simulink model "gm_sampleModel61442_pp_12_1_sub"  (R2023b)
settings: Solver=VariableStepAuto  StartTime=0.0  StopTime=10.0  RelTol=1e-3
libraries: simulink x37
(part 2 of 2)

== system gm_sampleModel61442_pp_12_1_sub/Subsystem/cfblk71 ==
  emi_243 : Inport  OutDataTypeStr=uint8  PortDimensions=1  SampleTime=1
  Action Port : Inport  Port=2  OutDataTypeStr=boolean  SampleTime=1
  Reshape : Reshape
  cfblk71_out1bypassMux : MultiPortSwitch  DataPortOrder=Zero-based contiguous  Inputs=2  zeroidx=on  OutDataTypeStr=uint8  SampleTime=1  SaturateOnIntegerOverflow=off  InputSameDT=off
  emi_244_bypass : UnitDelay  InitialCondition="fi(0,0,8,0,\"hex\",\"00\")"  SampleTime=1
  emi_244 : Outport  SampleTime=1  InitialOutput=0
  wires:
  Action Port/1 -> cfblk71_out1bypassMux/1
  emi_243/1 -> Reshape/1
  Reshape/1 -> cfblk71_out1bypassMux/3
  cfblk71_out1bypassMux/1 -> emi_244_bypass/1, emi_244/1
  emi_244_bypass/1 -> cfblk71_out1bypassMux/2

== system gm_sampleModel61442_pp_12_1_sub/Subsystem/cfblk72 ==
  emi_251 : Inport  OutDataTypeStr=uint8  PortDimensions=1  SampleTime=1
  Action Port : Inport  Port=2  OutDataTypeStr=boolean  SampleTime=1
  cfblk72 : MinMax
  cfblk72_out1bypassMux : MultiPortSwitch  DataPortOrder=Zero-based contiguous  Inputs=2  zeroidx=on  OutDataTypeStr=uint8  SampleTime=1  SaturateOnIntegerOverflow=off  InputSameDT=off
  emi_252_bypass : UnitDelay  InitialCondition="fi(0,0,8,0,\"hex\",\"00\")"  SampleTime=1
  emi_252 : Outport  SampleTime=1  InitialOutput=0
  wires:
  Action Port/1 -> cfblk72_out1bypassMux/1
  emi_251/1 -> cfblk72/1
  cfblk72/1 -> cfblk72_out1bypassMux/3
  cfblk72_out1bypassMux/1 -> emi_252_bypass/1, emi_252/1
  emi_252_bypass/1 -> cfblk72_out1bypassMux/2

== system gm_sampleModel61442_pp_12_1_sub/Subsystem/cfblk75_inst ==
  in1 : Inport  OutDataTypeStr=uint8  SampleTime=1
  in2 : Inport  Port=2  OutDataTypeStr=uint8  SampleTime=1
  mul_cfblk75_dotp_mulcomp : Product  Inputs=**  OutDataTypeStr=uint8  SampleTime=1
  out1 : Outport  OutDataTypeStr=uint8  SampleTime=1
  wires:
  in1/1 -> mul_cfblk75_dotp_mulcomp/1
  in2/1 -> mul_cfblk75_dotp_mulcomp/2
  mul_cfblk75_dotp_mulcomp/1 -> out1/1

== system gm_sampleModel61442_pp_12_1_sub/Subsystem/cfblk77 ==
  emi_259 : Inport  OutDataTypeStr=uint8  PortDimensions=1  SampleTime=1
  Action Port : Inport  Port=2  OutDataTypeStr=boolean  SampleTime=1
  cfblk77 : Subsystem  mask(Real World Value Increment){}
      mask help: Simulink:masks:RealWorldValueIncrement_MD
      mask Display: disp('V++')
  cfblk77_out1bypassMux : MultiPortSwitch  DataPortOrder=Zero-based contiguous  Inputs=2  zeroidx=on  OutDataTypeStr=uint8  SampleTime=1  SaturateOnIntegerOverflow=off  InputSameDT=off
  emi_260_bypass : UnitDelay  InitialCondition="fi(0,0,8,0,\"hex\",\"00\")"  SampleTime=1
  emi_260 : Outport  SampleTime=1  InitialOutput=0
  wires:
  Action Port/1 -> cfblk77_out1bypassMux/1
  emi_259/1 -> cfblk77/1(u)
  cfblk77/1(y) -> cfblk77_out1bypassMux/3
  cfblk77_out1bypassMux/1 -> emi_260_bypass/1, emi_260/1
  emi_260_bypass/1 -> cfblk77_out1bypassMux/2

== system gm_sampleModel61442_pp_12_1_sub/Subsystem/cfblk78 ==
  emi_131 : Inport  OutDataTypeStr=uint8  PortDimensions=1  SampleTime=1
  Action Port : Inport  Port=2  OutDataTypeStr=boolean  SampleTime=1
  cfblk78 : Signum  SampleTime=1
  cfblk78_out1bypassMux : MultiPortSwitch  DataPortOrder=Zero-based contiguous  Inputs=2  zeroidx=on  OutDataTypeStr=uint8  SampleTime=1  SaturateOnIntegerOverflow=off  InputSameDT=off
  emi_132_bypass : UnitDelay  InitialCondition="fi(0,0,8,0,\"hex\",\"00\")"  SampleTime=1
  emi_132 : Outport  SampleTime=1  InitialOutput=0
  wires:
  Action Port/1 -> cfblk78_out1bypassMux/1
  emi_131/1 -> cfblk78/1
  cfblk78/1 -> cfblk78_out1bypassMux/3
  cfblk78_out1bypassMux/1 -> emi_132_bypass/1, emi_132/1
  emi_132_bypass/1 -> cfblk78_out1bypassMux/2

== system gm_sampleModel61442_pp_12_1_sub/Subsystem/cfblk79 ==
  emi_267 : Inport  OutDataTypeStr=uint8  PortDimensions=1  SampleTime=1
  Action Port : Inport  Port=2  OutDataTypeStr=boolean  SampleTime=1
  cfblk79 : MinMax
  cfblk79_out1bypassMux : MultiPortSwitch  DataPortOrder=Zero-based contiguous  Inputs=2  zeroidx=on  OutDataTypeStr=uint8  SampleTime=1  SaturateOnIntegerOverflow=off  InputSameDT=off
  emi_268_bypass : UnitDelay  InitialCondition="fi(0,0,8,0,\"hex\",\"00\")"  SampleTime=1
  emi_268 : Outport  SampleTime=1  InitialOutput=0
  wires:
  Action Port/1 -> cfblk79_out1bypassMux/1
  emi_267/1 -> cfblk79/1
  cfblk79/1 -> cfblk79_out1bypassMux/3
  cfblk79_out1bypassMux/1 -> emi_268_bypass/1, emi_268/1
  emi_268_bypass/1 -> cfblk79_out1bypassMux/2

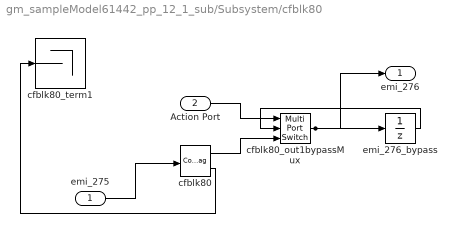
== system gm_sampleModel61442_pp_12_1_sub/Subsystem/cfblk80 ==
  emi_275 : Inport  OutDataTypeStr=uint8  PortDimensions=1  SampleTime=1
  Action Port : Inport  Port=2  OutDataTypeStr=boolean  SampleTime=1
  cfblk80 : ComplexToRealImag  SampleTime=1
  cfblk80_out1bypassMux : MultiPortSwitch  DataPortOrder=Zero-based contiguous  Inputs=2  zeroidx=on  OutDataTypeStr=uint8  SampleTime=1  SaturateOnIntegerOverflow=off  InputSameDT=off
  cfblk80_term1 : Terminator
  emi_276_bypass : UnitDelay  InitialCondition="fi(0,0,8,0,\"hex\",\"00\")"  SampleTime=1
  emi_276 : Outport  SampleTime=1  InitialOutput=0
  wires:
  Action Port/1 -> cfblk80_out1bypassMux/1
  emi_275/1 -> cfblk80/1
  cfblk80/1 -> cfblk80_out1bypassMux/3
  cfblk80/2 -> cfblk80_term1/1
  cfblk80_out1bypassMux/1 -> emi_276_bypass/1, emi_276/1
  emi_276_bypass/1 -> cfblk80_out1bypassMux/2

== system gm_sampleModel61442_pp_12_1_sub/Subsystem/cfblk81 ==
  emi_284 : Inport  OutDataTypeStr=uint8  PortDimensions=1  SampleTime=1
  Action Port : Inport  Port=2  OutDataTypeStr=boolean  SampleTime=1
  cfblk81 : MinMax
  cfblk81_out1bypassMux : MultiPortSwitch  DataPortOrder=Zero-based contiguous  Inputs=2  zeroidx=on  OutDataTypeStr=uint8  SampleTime=1  SaturateOnIntegerOverflow=off  InputSameDT=off
  emi_285_bypass : UnitDelay  InitialCondition="fi(0,0,8,0,\"hex\",\"00\")"  SampleTime=1
  emi_285 : Outport  SampleTime=1  InitialOutput=0
  wires:
  Action Port/1 -> cfblk81_out1bypassMux/1
  emi_284/1 -> cfblk81/1
  cfblk81/1 -> cfblk81_out1bypassMux/3
  cfblk81_out1bypassMux/1 -> emi_285_bypass/1, emi_285/1
  emi_285_bypass/1 -> cfblk81_out1bypassMux/2

== system gm_sampleModel61442_pp_12_1_sub/Subsystem/cfblk84 ==
  u : Inport  OutDataTypeStr=uint8  SampleTime=1
  FixPt Constant : Constant  DisableCoverage=on  OutDataTypeStr=Inherit: Inherit via back propagation  SampleTime=-1
  FixPt Data Type Duplicate : DataTypeDuplicate  DisableCoverage=on  NumInputPorts=3
  FixPt Sum1 : Sum  OutDataTypeStr=Inherit: Inherit via back propagation  InputSameDT=on  LockScale=on
  y : Outport  SampleTime=1
  wires:
  u/1 -> FixPt Sum1/1, FixPt Data Type Duplicate/2
  FixPt Constant/1 -> FixPt Sum1/2, FixPt Data Type Duplicate/3
  FixPt Sum1/1 -> FixPt Data Type Duplicate/1, y/1

== system gm_sampleModel61442_pp_12_1_sub/Subsystem/cfblk8_inst ==
  in1 : Inport  OutDataTypeStr=uint8  SampleTime=1
  in2 : Inport  Port=2  OutDataTypeStr=uint8  SampleTime=1
  mul_cfblk8_dotp_mulcomp : Product  Inputs=**  OutDataTypeStr=uint8  SampleTime=1
  out1 : Outport  OutDataTypeStr=uint8  SampleTime=1
  wires:
  in1/1 -> mul_cfblk8_dotp_mulcomp/1
  in2/1 -> mul_cfblk8_dotp_mulcomp/2
  mul_cfblk8_dotp_mulcomp/1 -> out1/1

== system gm_sampleModel61442_pp_12_1_sub/Subsystem/cfblk91 ==
  u : Inport  OutDataTypeStr=uint8  SampleTime=1
  FixPt Constant : Constant  DisableCoverage=on  OutDataTypeStr=Inherit: Inherit via back propagation  SampleTime=-1
  FixPt Data Type Duplicate : DataTypeDuplicate  DisableCoverage=on  NumInputPorts=3
  FixPt Sum1 : Sum  OutDataTypeStr=Inherit: Inherit via back propagation  InputSameDT=on  LockScale=on
  y : Outport  SampleTime=1
  wires:
  u/1 -> FixPt Sum1/1, FixPt Data Type Duplicate/2
  FixPt Constant/1 -> FixPt Sum1/2, FixPt Data Type Duplicate/3
  FixPt Sum1/1 -> FixPt Data Type Duplicate/1, y/1

== system gm_sampleModel61442_pp_12_1_sub/Subsystem/cfblk94_inst ==
  in1 : Inport  OutDataTypeStr=uint8  SampleTime=1
  in2 : Inport  Port=2  OutDataTypeStr=uint8  SampleTime=1
  mul_cfblk94_dotp_mulcomp : Product  Inputs=**  OutDataTypeStr=uint8  SampleTime=1
  out1 : Outport  OutDataTypeStr=uint8  SampleTime=1
  wires:
  in1/1 -> mul_cfblk94_dotp_mulcomp/1
  in2/1 -> mul_cfblk94_dotp_mulcomp/2
  mul_cfblk94_dotp_mulcomp/1 -> out1/1

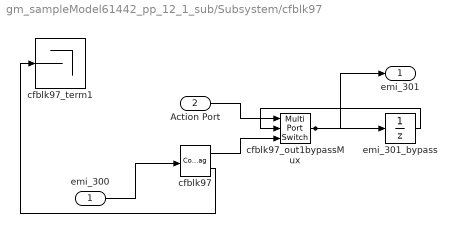
== system gm_sampleModel61442_pp_12_1_sub/Subsystem/cfblk97 ==
  emi_300 : Inport  OutDataTypeStr=uint8  PortDimensions=1  SampleTime=1
  Action Port : Inport  Port=2  OutDataTypeStr=boolean  SampleTime=1
  cfblk97 : ComplexToRealImag  SampleTime=1
  cfblk97_out1bypassMux : MultiPortSwitch  DataPortOrder=Zero-based contiguous  Inputs=2  zeroidx=on  OutDataTypeStr=uint8  SampleTime=1  SaturateOnIntegerOverflow=off  InputSameDT=off
  cfblk97_term1 : Terminator
  emi_301_bypass : UnitDelay  InitialCondition="fi(0,0,8,0,\"hex\",\"00\")"  SampleTime=1
  emi_301 : Outport  SampleTime=1  InitialOutput=0
  wires:
  Action Port/1 -> cfblk97_out1bypassMux/1
  emi_300/1 -> cfblk97/1
  cfblk97/1 -> cfblk97_out1bypassMux/3
  cfblk97/2 -> cfblk97_term1/1
  cfblk97_out1bypassMux/1 -> emi_301_bypass/1, emi_301/1
  emi_301_bypass/1 -> cfblk97_out1bypassMux/2

== system gm_sampleModel61442_pp_12_1_sub/Subsystem/cfblk1/cfblk1 ==
  note: Edge
  note: U(k)
  U : Inport  OutDataTypeStr=uint8  SampleTime=1
  Action Port_out2 : Inport  Port=2  OutDataTypeStr=boolean  SampleTime=1
  Delay Input1 : Subsystem
      settings: MinAlgLoopOccurrences=on
  FixPt Relational Operator : RelationalOperator  Operator=<  OutDataTypeStr=fixdt(0,8,0)  SampleTime=1  InputSameDT=off
  Y : Outport  SampleTime=1  InitialOutput=0
  wires:
  U/1 -> FixPt Relational Operator/1, Delay Input1/1(in0)
  Delay Input1/1(out0) -> FixPt Relational Operator/2
  FixPt Relational Operator/1 -> Y/1
  Action Port_out2/1 -> Delay Input1/Enable

== system gm_sampleModel61442_pp_12_1_sub/Subsystem/cfblk119/cfblk119 ==
  u : Inport  OutDataTypeStr=uint8  SampleTime=1
  FixPt Constant : Constant  DisableCoverage=on  OutDataTypeStr=Inherit: Inherit via back propagation  SampleTime=-1
  FixPt Data Type Duplicate : DataTypeDuplicate  DisableCoverage=on  NumInputPorts=3
  FixPt Sum1 : Sum  OutDataTypeStr=Inherit: Inherit via back propagation  InputSameDT=on  LockScale=on
  y : Outport  SampleTime=1  InitialOutput=0
  wires:
  u/1 -> FixPt Sum1/1, FixPt Data Type Duplicate/2
  FixPt Constant/1 -> FixPt Sum1/2, FixPt Data Type Duplicate/3
  FixPt Sum1/1 -> FixPt Data Type Duplicate/1, y/1

== system gm_sampleModel61442_pp_12_1_sub/Subsystem/cfblk168/cfblk168 ==
  in0 : Inport  OutDataTypeStr=uint8  SampleTime=1
  Action Port_out2 : EnablePort  OutDataTypeStr=boolean
  cfblk168 : Delay  DelayLength=double(2)  InitialCondition=0
  out0 : Outport  OutDataTypeStr=uint8  SampleTime=1  InitialOutput=0
  wires:
  cfblk168/1 -> out0/1
  in0/1 -> cfblk168/1

== system gm_sampleModel61442_pp_12_1_sub/Subsystem/cfblk2/cfblk2 ==
  note: U(k)
  note: Edge
  U : Inport  OutDataTypeStr=uint8  SampleTime=1
  Action Port_out2 : Inport  Port=2  OutDataTypeStr=boolean  SampleTime=1
  Delay Input1 : Subsystem
      settings: MinAlgLoopOccurrences=on
  FixPt Relational Operator : RelationalOperator  Operator=>  OutDataTypeStr=fixdt(0,8,0)  SampleTime=1  InputSameDT=off
  Positive : Subsystem  mask(Compare To Zero){relop=>, OutDataTypeStr=boolean, ZeroCross=off}
      mask prompts: relop "Simulink:masks:Operator_MP"; OutDataTypeStr "Simulink:masks:OutputDataType_MP"; ZeroCross "Simulink:masks:EnableZerocrossingDetection_MP"
      mask help: Simulink:masks:CompareToZero_MD
      mask TypeOptions relop: == | ~= | < | <= | >= | >
      mask TypeOptions OutDataTypeStr: Simulink:masks:uint8 | Simulink:masks:boolean
      mask Callback ZeroCross: sl('zeroCrossEnable', gcbh);
      mask Display: disp([relop,' 0'])
  Y : Outport  SampleTime=1  InitialOutput=0
  wires:
  U/1 -> Positive/1(u)
  Delay Input1/1(out0) -> FixPt Relational Operator/2
  FixPt Relational Operator/1 -> Y/1
  Positive/1(y) -> FixPt Relational Operator/1, Delay Input1/1(in0)
  Action Port_out2/1 -> Delay Input1/Enable

== system gm_sampleModel61442_pp_12_1_sub/Subsystem/cfblk28/cfblk28 ==
  u : Inport  OutDataTypeStr=uint8  SampleTime=1
  FixPt Constant : Constant  DisableCoverage=on  OutDataTypeStr=Inherit: Inherit via back propagation  SampleTime=-1
  FixPt Data Type Duplicate : DataTypeDuplicate  DisableCoverage=on  NumInputPorts=3
  FixPt Sum1 : Sum  OutDataTypeStr=Inherit: Inherit via back propagation  InputSameDT=on  LockScale=on
  y : Outport  SampleTime=1  InitialOutput=0
  wires:
  u/1 -> FixPt Sum1/1, FixPt Data Type Duplicate/2
  FixPt Constant/1 -> FixPt Sum1/2, FixPt Data Type Duplicate/3
  FixPt Sum1/1 -> FixPt Data Type Duplicate/1, y/1

== system gm_sampleModel61442_pp_12_1_sub/Subsystem/cfblk3/cfblk3 ==
  note: Edge
  note: U(k)
  U : Inport  OutDataTypeStr=uint8  SampleTime=1
  Action Port_out2 : Inport  Port=2  OutDataTypeStr=boolean  SampleTime=1
  Delay Input1 : Subsystem
      settings: MinAlgLoopOccurrences=on
  FixPt Relational Operator : RelationalOperator  Operator=~=  OutDataTypeStr=fixdt(0,8,0)  SampleTime=1  InputSameDT=off
  Y : Outport  SampleTime=1  InitialOutput=0
  wires:
  U/1 -> FixPt Relational Operator/1, Delay Input1/1(in0)
  Delay Input1/1(out0) -> FixPt Relational Operator/2
  FixPt Relational Operator/1 -> Y/1
  Action Port_out2/1 -> Delay Input1/Enable

== system gm_sampleModel61442_pp_12_1_sub/Subsystem/cfblk77/cfblk77 ==
  u : Inport  OutDataTypeStr=uint8  SampleTime=1
  FixPt Constant : Constant  DisableCoverage=on  OutDataTypeStr=Inherit: Inherit via back propagation  SampleTime=-1
  FixPt Data Type Duplicate : DataTypeDuplicate  DisableCoverage=on  NumInputPorts=3
  FixPt Sum1 : Sum  OutDataTypeStr=Inherit: Inherit via back propagation  InputSameDT=on  LockScale=on
  y : Outport  SampleTime=1  InitialOutput=0
  wires:
  u/1 -> FixPt Sum1/1, FixPt Data Type Duplicate/2
  FixPt Constant/1 -> FixPt Sum1/2, FixPt Data Type Duplicate/3
  FixPt Sum1/1 -> FixPt Data Type Duplicate/1, y/1

== system gm_sampleModel61442_pp_12_1_sub/Subsystem/cfblk1/cfblk1/Delay Input1 ==
  in0 : Inport  OutDataTypeStr=uint8  SampleTime=1
  Action Port_out2 : EnablePort  OutDataTypeStr=boolean
  Delay Input1 : Delay  DelayLength=double(1)  InitialCondition=0
  out0 : Outport  OutDataTypeStr=uint8  SampleTime=1  InitialOutput=0
  wires:
  Delay Input1/1 -> out0/1
  in0/1 -> Delay Input1/1

== system gm_sampleModel61442_pp_12_1_sub/Subsystem/cfblk2/cfblk2/Delay Input1 ==
  in0 : Inport  OutDataTypeStr=boolean  SampleTime=1
  Action Port_out2 : EnablePort  OutDataTypeStr=boolean
  Delay Input1 : UnitDelay  SampleTime=1
  out0 : Outport  OutDataTypeStr=boolean  SampleTime=1  InitialOutput=0
  wires:
  Delay Input1/1 -> out0/1
  in0/1 -> Delay Input1/1

== system gm_sampleModel61442_pp_12_1_sub/Subsystem/cfblk2/cfblk2/Positive ==
  u : Inport  OutDataTypeStr=uint8  SampleTime=1
  Compare : RelationalOperator  Operator=>  OutDataTypeStr=boolean  SampleTime=1
  Constant : Constant  Value=0  OutDataTypeStr=uint8  SampleTime=1
  y : Outport  SampleTime=1  InitialOutput=0
  wires:
  u/1 -> Compare/1
  Compare/1 -> y/1
  Constant/1 -> Compare/2

== system gm_sampleModel61442_pp_12_1_sub/Subsystem/cfblk3/cfblk3/Delay Input1 ==
  in0 : Inport  OutDataTypeStr=uint8  SampleTime=1
  Action Port_out2 : EnablePort  OutDataTypeStr=boolean
  Delay Input1 : Delay  DelayLength=double(1)  InitialCondition=0
  out0 : Outport  OutDataTypeStr=uint8  SampleTime=1  InitialOutput=0
  wires:
  Delay Input1/1 -> out0/1
  in0/1 -> Delay Input1/1
